simulink model "NMPChighFidelityTiltingQuadrotor"  (R2022b)
settings: Solver=ode4  StartTime=0.0  StopTime=15  FixedStep=Ts  RelTol=1e-3
InitFcn:
  | run initNMPChighFidelityTiltingQuadrotor.m
values from neighbouring files (symbols this model uses):
  lb = 0    [initNMPChighFidelityTiltingQuadrotor.m]
  lbu = repmat(lbu,1,N)    [initNMPChighFidelityTiltingQuadrotor.m]
  lbx = 0    [initNMPChighFidelityTiltingQuadrotor.m]
  N = 30    [initNMPChighFidelityTiltingQuadrotor.m]
  para = repmat(para0,1,N+1)    [initNMPChighFidelityTiltingQuadrotor.m]
  Ts_st = settings.Ts_st    [initNMPChighFidelityTiltingQuadrotor.m]
  ub = 0    [initNMPChighFidelityTiltingQuadrotor.m]
  ubu = repmat(ubu,1,N)    [initNMPChighFidelityTiltingQuadrotor.m]
  ubx = 0    [initNMPChighFidelityTiltingQuadrotor.m]
  W = repmat([Qp Qeq Qv Qomega Qalpha Qw_bar2 Qup Qdotalpha]',1, N)    [initNMPChighFidelityTiltingQuadrotor.m]
  WN = [Qp Qeq Qv Qomega Qalpha Qw_bar2]'    [initNMPChighFidelityTiltingQuadrotor.m]
  z0 = 0    [initNMPChighFidelityTiltingQuadrotor.m]
undefined symbols (not defined in the file or in its folder): DiscIntNeverNeededParam, opt, prop, rad, s, settings, tiltq
libraries: simulink_extras x3, slpidlib x2, aerolibconvert2 x1, robotcorelib x1, uavutilslib x1
settings Model: PauseTimes=2  Creator=chen  LastModifiedBy=beniamino
settings SolverCC: AlgebraicLoopSolver=TrustRegion
settings DataIOCC: ReturnWorkspaceOutputs=off
settings DebuggingCC: UnconnectedInputMsg=warning  UnconnectedOutputMsg=warning  UnconnectedLineMsg=warning  SFMachineParentedDataDiag=warning  ArithmeticOperatorsInVariantConditions=warning
settings ModelReferenceCC: EnableRefExpFcnMdlSchedulingChecks=on
settings SFSimCC: SimUseLocalCustomCode=off  CustomCodeUndefinedFunction=UseInterfaceOnly
settings RTWCC: RTWUseLocalCustomCode=off  CheckMdlBeforeBuild=Error

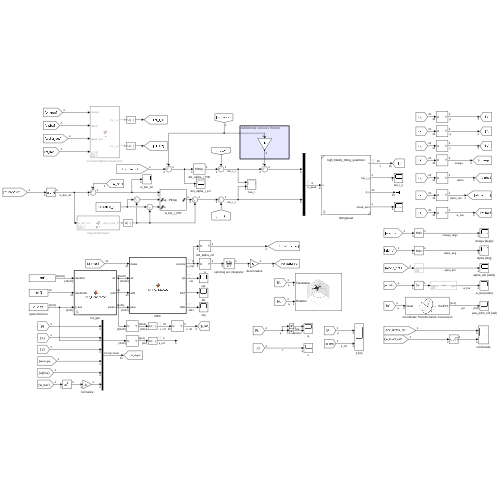
[thumbnail: Simulink's stored preview of the top-level diagram]
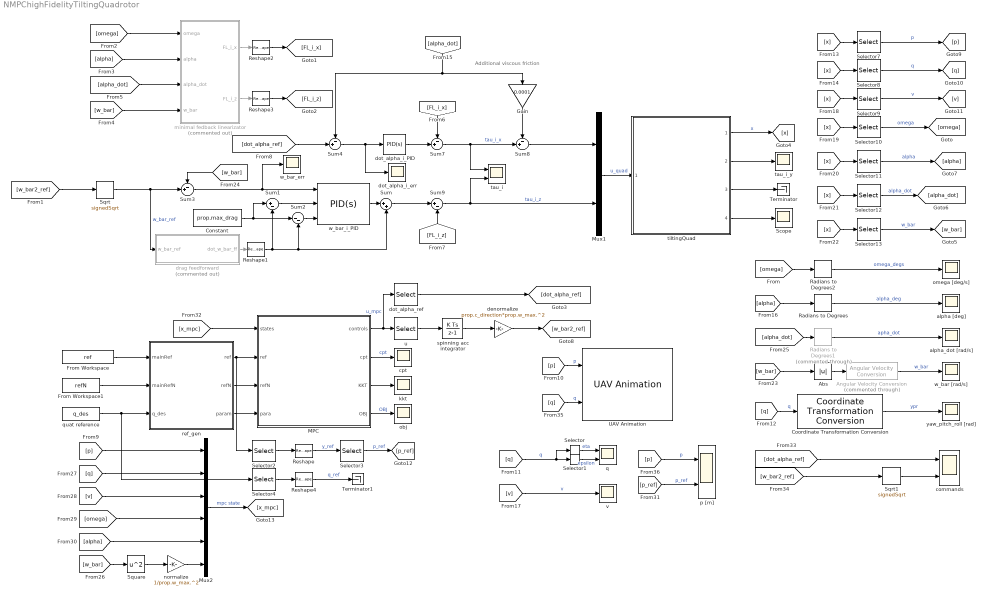
== system NMPChighFidelityTiltingQuadrotor ==
  note: Additional viscous friction
  Abs : Abs  SaturateOnIntegerOverflow=off
  Angular Velocity Conversion : aerolibconvert2/Angular Velocity Conversion  Commented=through  IU=rad/s  OU=rpm
  Constant : Constant  Value=prop.max_drag
  Coordinate Transformation Conversion : robotcorelib/Coordinate Transformation Conversion  InputRepresentation=Quaternion  InputEulerSequence=ZYX  ShowTrVecInputPort=on  OutputRepresentation=Euler Angles  OutputEulerSequence=ZYX  ShowTrVecOutputPort=on  SimulateUsing=Code generation
  From Workspace : FromWorkspace  VariableName=ref  SampleTime=Ts_st  Interpolate=off  OutputAfterFinalValue=Holding final value
  From Workspace1 : FromWorkspace  VariableName=refN  SampleTime=Ts_st  Interpolate=off  OutputAfterFinalValue=Holding final value
  Gain : Gain  Gain=0.0001
  MPC : MATLAB Function  TreatAsAtomicUnit=on
  Mux1 : Mux  Inputs=2
  Mux2 : Mux  Inputs=6
  Radians to Degrees : simulink_extras/Transformations/Radians to Degrees
  Radians to Degrees1 : simulink_extras/Transformations/Radians to Degrees  Commented=through
  Radians to Degrees2 : simulink_extras/Transformations/Radians to Degrees
  Reshape{,1..4} (5 alike) : Reshape
  Scope : Scope
  Selector : Selector  InputPortWidth=4  IndexOptions=Index vector (dialog)  Indices=1  OutputSizes=1
  Selector1 : Selector  InputPortWidth=4  IndexOptions=Index vector (dialog)  Indices=2:4  OutputSizes=1
  Selector10 : Selector  InputPortWidth=25  IndexOptions=Index vector (dialog)  Indices=11:13  OutputSizes=1
  Selector11 : Selector  InputPortWidth=25  IndexOptions=Index vector (dialog)  Indices=14:17  OutputSizes=1
  Selector12 : Selector  InputPortWidth=25  IndexOptions=Index vector (dialog)  Indices=18:21  OutputSizes=1
  Selector13 : Selector  InputPortWidth=25  IndexOptions=Index vector (dialog)  Indices=22:25  OutputSizes=1
  Selector2 : Selector  NumberOfDimensions=2  InputPortWidth=[27 N]  IndexOptions=Select all,Index vector (dialog)  Indices=1:3,1  OutputSizes=1,1
  Selector3 : Selector  InputPortWidth=28  IndexOptions=Index vector (dialog)  Indices=1:3  OutputSizes=1
  Selector4 : Selector  NumberOfDimensions=2  InputPortWidth=[27 N]  IndexOptions=Select all,Index vector (dialog)  Indices=1:3,1  OutputSizes=1,1
  Selector7 : Selector  InputPortWidth=25  IndexOptions=Index vector (dialog)  Indices=1:3  OutputSizes=1
  Selector8 : Selector  InputPortWidth=25  IndexOptions=Index vector (dialog)  Indices=4:7  OutputSizes=1
  Selector9 : Selector  InputPortWidth=25  IndexOptions=Index vector (dialog)  Indices=8:10  OutputSizes=1
  Sqrt : Sqrt  Operator=signedSqrt
  Sqrt1 : Sqrt  Operator=signedSqrt
  Square : Math  Operator=square
  Sum : Sum  Inputs=|++
  Sum1 : Sum  Inputs=|+-
  Sum2 : Sum  Inputs=|--
  Sum{3..4,7..8} (4 alike) : Sum  Inputs=-+|
  Sum9 : Sum  Inputs=|+-
  Terminator : Terminator
  Terminator1 : Terminator
  UAV Animation : uavutilslib/UAV Animation  UAVType=Multirotor  UAVSize=1  InertialZDirection=Up  SampleTime=0.02
  alpha [deg] : Scope
  alpha_dot [rad/s] : Scope
  commands : Scope  NumInputPorts=2
  cpt : Scope
  denormalize : Gain  Gain=prop.c_direction*prop.w_max.^2
  dot_alpha_i_PID : slpidlib/PID Controller  Controller=PID  Form=Parallel  TimeDomain=Continuous-time  UseExternalTs=off  SampleTime=-1  IntegratorMethod=Forward Euler  FilterMethod=Forward Euler  ControllerParametersSource=internal  P=0.01  I=0.1  UseKiTs=off  D=0.00001  N=100  UseFilter=on  TunerSelectOption=Transfer Function Based (PID Tuner App)  InitialConditionSource=internal  InitialConditionForIntegrator=0  InitialConditionForFilter=0  DifferentiatorICPrevScaledInput=0  ExternalReset=none  TrackingMode=off  Kt=1  LimitOutput=off  SatLimitsSource=internal  UpperSaturationLimit=inf  LowerSaturationLimit=-inf  LinearizeAsGain=on  AntiWindupMode=none  Kb=1  LimitIntegrator=off  UpperIntegratorSaturationLimit=inf  LowerIntegratorSaturationLimit=-inf  POutMin=[]  POutMax=[]  IOutMin=[]  IOutMax=[]  DOutMin=[]  DOutMax=[]  NOutMin=[]  NOutMax=[]  SumOutMin=[]  SumOutMax=[]  SaturationOutMin=[]  SaturationOutMax=[]  PParamMin=[]  PParamMax=[]  IParamMin=[]  IParamMax=[]  DParamMin=[]  DParamMax=[]  NParamMin=[]  NParamMax=[]  KbParamMin=[]  KbParamMax=[]  KtParamMin=[]  KtParamMax=[]  KbOutMin=[]  KbOutMax=[]  KtOutMin=[]  KtOutMax=[]  IntegratorOutMin=[]  IntegratorOutMax=[]  FilterOutMin=[]  FilterOutMax=[]  SumI1OutMin=[]  SumI1OutMax=[]  SumI2OutMin=[]  SumI2OutMax=[]  SumI3OutMin=[]  SumI3OutMax=[]  SumI4OutMin=[]  SumI4OutMax=[]  SumDOutMin=[]  SumDOutMax=[]  DifferentiatorOutMin=[]  DifferentiatorOutMax=[]  FilterDiffOutCoefMin=[]  FilterDiffOutCoefMax=[]  ReciprocalOutMin=[]  ReciprocalOutMax=[]  SumDenOutMin=[]  SumDenOutMax=[]  SumNumOutMin=[]  SumNumOutMax=[]  DivideOutMin=[]  DivideOutMax=[]  UdiffTsProdOutMin=[]  UdiffTsProdOutMax=[]  NTsProdOutMin=[]  NTsProdOutMax=[]  UintegralTsProdOutMin=[]  UintegralTsProdOutMax=[]  UngainTsProdOutMin=[]  UngainTsProdOutMax=[]  ClampingZeroOutDataTypeStr=Inherit: Inherit via back propagation  ClampingZeroOutMin=[]  ClampingZeroOutMax=[]  FilterDenConstantOutDataTypeStr=Inherit: Inherit via back propagation  FilterDenConstantOutMin=[]  FilterDenConstantOutMax=[]  PCopyOutDataTypeStr=Inherit: Inherit via back propagation  PCopyOutMin=[]  PCopyOutMax=[]  NCopyOutDataTypeStr=Inherit: Inherit via back propagation  NCopyOutMin=[]  NCopyOutMax=[]  IntegratorContinuousStateAttributes=''  IntegratorStateMustResolveToSignalObject=off  IntegratorRTWStateStorageClass=Auto  FilterContinuousStateAttributes=''  FilterStateMustResolveToSignalObject=off  FilterRTWStateStorageClass=Auto  ParallelPVariant=InternalParameters  IdealPVariant=Disabled  IVariant=InternalParameters  DVariant=InternalParameters  IntegratorVariant=Continuous  SatVariant=Disabled  AWVariant=Passthrough  PCopyVariant=Disabled  TRVariant=Disabled  FdbkBlocksVariant=Forward  IdealPFdbkVariant=Disabled  SatFdbkVariant=Disabled  DerivativeFilterVariant=ContFilter  NVariant=InternalParameters  NCopyVariant=Disabled  FilterICVariant=InternalICsFilter  IntegratorICVariant=InternalICs  ExternalResetVariant=Disabled  TRSumVariant=Passthrough  SumFdbkVariant=Disabled  SumVariant=Sum_PID  TsampFilterVariant=InternalTs  TsampNgainVariant=Passthrough  TsampIntegralVariant=Passthrough  ExternalSaturationOutDataTypeStr=Inherit: Same as second input
  dot_alpha_i_err : Scope
  dot_alpha_ref : Selector  InputPortWidth=8  IndexOptions=Index vector (dialog)  Indices=5:8  OutputSizes=1
  drag feedforward : MATLAB Function  Commented=on  TreatAsAtomicUnit=on  mask{k_m=prop.k_m}
      mask prompts: k_m "motor drag constant"
  kkt : Scope
  minimal fedback linearizator : MATLAB Function  Commented=on  TreatAsAtomicUnit=on  mask{N=tiltq.N, I_i=tiltq.I_i, beta=tiltq.beta}
      mask prompts: N "number of propellers"; I_i "propeller + rotor inertia matrix"; beta "propeller tilting planes angles"
  normalize : Gain  Gain=1/prop.w_max.^2
  obj : Scope
  omega [deg/s] : Scope
  p [m] : Scope  NumInputPorts=2
  q : Scope  NumInputPorts=2
  quat reference : FromWorkspace  VariableName=q_des  SampleTime=Ts_st  Interpolate=off  OutputAfterFinalValue=Holding final value
  ref_gen : MATLAB Function  TreatAsAtomicUnit=on  mask{opt=opt}
      mask prompts: opt "Simulations options structure"
  spinning acc integrator : DiscreteIntegrator  InitialCondition=0.33*ones(4,1)  SampleTime=-1  ICPrevOutput=DiscIntNeverNeededParam  ICPrevScaledInput=DiscIntNeverNeededParam
  tau_i : Scope  NumInputPorts=2
  tau_i_y : Scope
  tiltingQuad : Subsystem  ReferencedSubsystem=high_fidelity_tilting_quadrotor  p0=p_0  q0=q_0  v0=v_0  omega0=omega_0  alpha0=alpha_0  d_alpha_0=alpha_dot_0  bar_w0=w_bar_0  m_b=tiltq.m_b  beta=tiltq.beta  I_b=body.I  I_i=tiltq.I_i  c_direction=prop.c_direction  k_m=prop.k_m  k_t=prop.k_t  p_mot=tiltq.p_mot  min_alpha=tiltq.min_alpha  max_alpha=tiltq.max_alpha  min_d_alpha=tiltq.min_alpha_dot  max_d_alpha=tiltq.max_alpha_dot  min_bar_w=[prop.w_min prop.w_min -prop.w_max -prop.w_max]  max_bar_w=[prop.w_max prop.w_max -prop.w_min -prop.w_min]
  u : Selector  InputPortWidth=8  IndexOptions=Index vector (dialog)  Indices=1:4  OutputSizes=1
  v : Scope
  w_bar [rad/s] : Scope
  w_bar_err : Scope
  w_bar_i_PID : slpidlib/PID Controller  Controller=PID  Form=Parallel  TimeDomain=Continuous-time  UseExternalTs=off  SampleTime=-1  IntegratorMethod=Forward Euler  FilterMethod=Forward Euler  ControllerParametersSource=internal  P=0.01  I=0.1  UseKiTs=on  D=0.00001  N=100  UseFilter=on  TunerSelectOption=Transfer Function Based (PID Tuner App)  InitialConditionSource=internal  InitialConditionForIntegrator=0  InitialConditionForFilter=0  DifferentiatorICPrevScaledInput=0  ExternalReset=none  TrackingMode=off  Kt=1  LimitOutput=on  SatLimitsSource=external  UpperSaturationLimit=inf  LowerSaturationLimit=-inf  LinearizeAsGain=on  AntiWindupMode=back-calculation  Kb=10  LimitIntegrator=off  UpperIntegratorSaturationLimit=inf  LowerIntegratorSaturationLimit=-inf  POutMin=[]  POutMax=[]  IOutMin=[]  IOutMax=[]  DOutMin=[]  DOutMax=[]  NOutMin=[]  NOutMax=[]  SumOutMin=[]  SumOutMax=[]  SaturationOutMin=[]  SaturationOutMax=[]  PParamMin=[]  PParamMax=[]  IParamMin=[]  IParamMax=[]  DParamMin=[]  DParamMax=[]  NParamMin=[]  NParamMax=[]  KbParamMin=[]  KbParamMax=[]  KtParamMin=[]  KtParamMax=[]  KbOutMin=[]  KbOutMax=[]  KtOutMin=[]  KtOutMax=[]  IntegratorOutMin=[]  IntegratorOutMax=[]  FilterOutMin=[]  FilterOutMax=[]  SumI1OutMin=[]  SumI1OutMax=[]  SumI2OutMin=[]  SumI2OutMax=[]  SumI3OutMin=[]  SumI3OutMax=[]  SumI4OutMin=[]  SumI4OutMax=[]  SumDOutMin=[]  SumDOutMax=[]  DifferentiatorOutMin=[]  DifferentiatorOutMax=[]  FilterDiffOutCoefMin=[]  FilterDiffOutCoefMax=[]  ReciprocalOutMin=[]  ReciprocalOutMax=[]  SumDenOutMin=[]  SumDenOutMax=[]  SumNumOutMin=[]  SumNumOutMax=[]  DivideOutMin=[]  DivideOutMax=[]  UdiffTsProdOutMin=[]  UdiffTsProdOutMax=[]  NTsProdOutMin=[]  NTsProdOutMax=[]  UintegralTsProdOutMin=[]  UintegralTsProdOutMax=[]  UngainTsProdOutMin=[]  UngainTsProdOutMax=[]  ClampingZeroOutDataTypeStr=Inherit: Inherit via back propagation  ClampingZeroOutMin=[]  ClampingZeroOutMax=[]  FilterDenConstantOutDataTypeStr=Inherit: Inherit via back propagation  FilterDenConstantOutMin=[]  FilterDenConstantOutMax=[]  PCopyOutDataTypeStr=Inherit: Inherit via back propagation  PCopyOutMin=[]  PCopyOutMax=[]  NCopyOutDataTypeStr=Inherit: Inherit via back propagation  NCopyOutMin=[]  NCopyOutMax=[]  IntegratorContinuousStateAttributes=''  IntegratorStateMustResolveToSignalObject=off  IntegratorRTWStateStorageClass=Auto  FilterContinuousStateAttributes=''  FilterStateMustResolveToSignalObject=off  FilterRTWStateStorageClass=Auto  ParallelPVariant=InternalParameters  IdealPVariant=Disabled  IVariant=InternalParameters  DVariant=InternalParameters  IntegratorVariant=Continuous  SatVariant=External  AWVariant=BackCalculation  PCopyVariant=Disabled  TRVariant=Disabled  FdbkBlocksVariant=Forward  IdealPFdbkVariant=Disabled  SatFdbkVariant=Disabled  DerivativeFilterVariant=ContFilter  NVariant=InternalParameters  NCopyVariant=Disabled  FilterICVariant=InternalICsFilter  IntegratorICVariant=InternalICs  ExternalResetVariant=Disabled  TRSumVariant=Passthrough  SumFdbkVariant=Disabled  SumVariant=Sum_PID  TsampFilterVariant=InternalTs  TsampNgainVariant=Passthrough  TsampIntegralVariant=Passthrough  ExternalSaturationOutDataTypeStr=Inherit: Same as second input
  yaw_pitch_roll [rad] : Scope
  wires:
  MPC/1(controls) -> u/1, dot_alpha_ref/1  "u_mpc"
  MPC/2(cpt) -> cpt/1  "cpt"
  MPC/4(OBJ) -> obj/1  "OBJ"
  MPC/3(KKT) -> kkt/1
  ref_gen/1(ref) -> Selector2/1, MPC/2(ref)
  ref_gen/2(refN) -> MPC/3(refN)
  [alpha_dot] -> Sum4/1, Gain/1
  Mux1/1 -> tiltingQuad/1  "u_quad"
  Sum2/1 -> w_bar_i_PID/3
  [w_bar] -> minimal fedback linearizator/4(w_bar)
  Reshape1/1 -> Sum/2, Sum2/2, Sum1/2
  Gain/1 -> Sum8/1
  tiltingQuad/3 -> Terminator/1
  [w_bar] -> Sum3/1
  minimal fedback linearizator/1(FL_i_x) -> Reshape2/1
  tiltingQuad/1 -> [x]  "x"
  tiltingQuad/2 -> tau_i_y/1
  Sum7/1 -> tau_i/1, Sum8/2  "tau_i_x"
  Sum1/1 -> w_bar_i_PID/2
  [omega] -> minimal fedback linearizator/1(omega)
  Sum9/1 -> Mux1/2, tau_i/2  "tau_i_z"
  [w_bar2_ref] -> Sqrt/1
  [FL_i_x] -> Sum7/1
  [FL_i_z] -> Sum9/2
  w_bar_i_PID/1 -> Sum/1
  Constant/1 -> Sum2/1, Sum1/1
  [alpha_dot] -> minimal fedback linearizator/3(alpha_dot)
  tiltingQuad/4 -> Scope/1
  Sum4/1 -> dot_alpha_i_err/1, dot_alpha_i_PID/1
  [alpha] -> minimal fedback linearizator/2(alpha)
  minimal fedback linearizator/2(FL_i_z) -> Reshape3/1
  Sum8/1 -> Mux1/1
  Sum/1 -> Sum9/1
  Sqrt/1 -> Sum3/2, drag feedforward/1(w_bar_ref)  "w_bar_ref"
  dot_alpha_i_PID/1 -> Sum7/2
  [x] -> Selector10/1
  Selector11/1 -> [alpha]  "alpha"
  Selector12/1 -> [alpha_dot]  "alpha_dot"
  Selector10/1 -> [omega]  "omega"
  [x] -> Selector13/1
  Selector13/1 -> [w_bar]  "w_bar"
  [x] -> Selector12/1
  [x] -> Selector11/1
  [alpha] -> Radians to Degrees/1
  Selector1/1 -> q/2  "epsilon"
  Radians to Degrees/1 -> alpha [deg]/1  "alpha_deg"
  [q] -> Selector1/1, Selector/1  "q"
  Radians to Degrees2/1 -> omega [deg/s]/1  "omega_degs"
  Radians to Degrees1/1 -> alpha_dot [rad/s]/1  "apha_dot"
  [w_bar] -> Abs/1
  Angular Velocity Conversion/1 -> w_bar [rad/s]/1  "w_bar"
  [x] -> Selector9/1
  Abs/1 -> Angular Velocity Conversion/1
  [x] -> Selector8/1
  [alpha_dot] -> Radians to Degrees1/1
  [p] -> UAV Animation/1  "p"
  Selector/1 -> q/1  "eta"
  [omega] -> Radians to Degrees2/1
  [v] -> v/1  "v"
  [x] -> Selector7/1
  dot_alpha_ref/1 -> [dot_alpha_ref]
  u/1 -> spinning acc integrator/1
  denormalize/1 -> [w_bar2_ref]
  [dot_alpha_ref] -> Sum4/2
  Sqrt1/1 -> commands/2
  Coordinate Transformation Conversion/1 -> yaw_pitch_roll [rad]/1  "ypr"
  Mux2/1 -> [x_mpc]  "mpc state"
  [w_bar] -> Square/1
  Square/1 -> normalize/1
  normalize/1 -> Mux2/6
  Sum3/1 -> w_bar_err/1, w_bar_i_PID/1
  spinning acc integrator/1 -> denormalize/1
  Selector7/1 -> [p]  "p"
  Selector8/1 -> [q]  "q"
  [q] -> Coordinate Transformation Conversion/1  "q"
  Selector9/1 -> [v]  "v"
  [alpha] -> Mux2/5
  [omega] -> Mux2/4
  [v] -> Mux2/3
  [q] -> Mux2/2
  [p] -> Mux2/1
  From Workspace/1 -> ref_gen/1(mainRef)
  From Workspace1/1 -> ref_gen/2(mainRefN)
  quat reference/1 -> Selector4/1, ref_gen/3(q_des)
  ref_gen/3(param) -> MPC/4(para)
  Selector2/1 -> Reshape/1
  [p_ref] -> p [m]/2  "p_ref"
  Reshape/1 -> Selector3/1  "y_ref"
  drag feedforward/1(dot_w_bar_ff) -> Reshape1/1
  Reshape2/1 -> [FL_i_x]
  Reshape3/1 -> [FL_i_z]
  [x_mpc] -> MPC/1(states)
  [w_bar2_ref] -> Sqrt1/1
  [dot_alpha_ref] -> commands/1
  [q] -> UAV Animation/2  "q"
  [p] -> p [m]/1  "p"
  Selector3/1 -> [p_ref]  "p_ref"
  Selector4/1 -> Reshape4/1
  Reshape4/1 -> Terminator1/1  "q_ref"

== matlab function NMPChighFidelityTiltingQuadrotor/ref_gen ==
  data: ref output; settings parameter; refN output; mainRef input; opt parameter; mainRefN input; q_des input; param output; para parameter
function [ref,refN, param] = Ref_Generator(settings, mainRef, opt, mainRefN, q_des, para)

switch opt.ref_type
    case 0
        p_ref = [1 1 1];
        qe_ref = [0 0 0];
        v_ref = [0 0 0];
        omega_ref = [0 0 0];
        alpha_ref = [0 0 0 0];
        w_bar_ref = 0.33*ones(1,4);
        u_ref = [0 0 0 0];
        dot_alpha_ref = [0 0 0 0];
        REF=[p_ref qe_ref v_ref omega_ref alpha_ref w_bar_ref u_ref dot_alpha_ref];
        ref = repmat(REF',1,settings.N);
        refN = REF(1:settings.nyN)';
        param = para;
    case 2
        ref = mainRef;
        refN = mainRefN;
        param =  q_des;
    otherwise
        p_ref = [0 0 0];
        qe_ref = [0 0 0];
        v_ref = [0 0 0];
        omega_ref = [0 0 0];
        alpha_ref = [0 0 0 0];
        w_bar_ref = 0.33*ones(1,4);
        u_ref = [0 0 0 0];
        dot_alpha_ref = [0 0 0 0];
        REF=[p_ref qe_ref v_ref omega_ref alpha_ref w_bar_ref u_ref dot_alpha_ref];
        ref = repmat(REF',1,settings.N);
        refN = REF(1:settings.nyN)';
        param = para;
end


%     ref = repmat([1.4, 0, 0]',1,settings.N);
%     refN = 1.4;

== matlab function NMPChighFidelityTiltingQuadrotor/minimal fedback linearizator ==
  data: omega input; alpha input; FL_i_x output; beta parameter; N parameter; alpha_dot input; w_bar input; FL_i_z output; I_i parameter
function [FL_i_x, FL_i_z]= fcn(omega, alpha, beta, N, alpha_dot, w_bar, I_i)

FL_i_x = zeros(4,1);
FL_i_z = zeros(4,1);

for i=1:N
    B_R_i = axang2rotm([0 0 1 beta(i)])*axang2rotm([1 0 0 alpha(i)]);
    omega_i = B_R_i.' * omega + [alpha_dot(i); 0; w_bar(i)];
    coriol_i = cross(omega_i, I_i*omega_i);
    FF_i = coriol_i;
    FL_i_x(i) = -FF_i(1);
    FL_i_z(i) = -FF_i(3);
end

== matlab function NMPChighFidelityTiltingQuadrotor/drag feedforward ==
  data: w_bar_ref input; dot_w_bar_ff output; k_m parameter
function dot_w_bar_ff = fcn(w_bar_ref, k_m)

dot_w_bar_ff = k_m .* w_bar_ref .* abs(w_bar_ref);

== matlab function NMPChighFidelityTiltingQuadrotor/MPC ==
  settings: updateMethod=DISCRETE  sampleTime=Ts_st
  data: states input size=nx; settings parameter; opt parameter; lb parameter; ub parameter; lbx parameter; ubx parameter; lbu parameter; ubu parameter; W parameter; WN parameter; ref input size=[ny N]; refN input size=nyN; z0 parameter; controls output size=nu; cpt output size=1; KKT output; OBJ output; para input
function [controls, cpt, KKT, OBJ] = NMPC_BLOCK(states, settings, opt, lb, ub, lbx, ubx, lbu, ubu, W, WN, ref, refN, z0, para)

%% everything should has a fixed size
coder.extrinsic('mpc_nmpcsolver_simulink');  
coder.extrinsic('InitData');  
coder.extrinsic('InitMemory');  
coder.extrinsic('evalin');
coder.extrinsic('assignin');

%%

persistent x u z lambda mu mu_x mu_u;
persistent input mem;

if isempty(input)  
    
    nx = settings.nx;        % No. of differential states
    nu = settings.nu;        % No. of controls
    nz = settings.nz;        % No. of algebraic states
    ny = settings.ny;        % No. of outputs (references)    
    nyN= settings.nyN;       % No. of outputs at terminal stage 
    np = settings.np;        % No. of parameters (on-line data)
    nc = settings.nc;        % No. of constraints
    ncN = settings.ncN;      % No. of constraints at terminal stage
    nbu = settings.nbu;      % No. of control bounds
    nbx = settings.nbx;      % No. of state bounds
    nbu_idx = settings.nbu_idx; % Index of control bounds
    nbx_idx = settings.nbx_idx; % Index of state bounds
    N = settings.N;
    N2 = settings.N2;
    r = settings.r;
        
    input.x0=states;
    
    x=repmat(states,1,N+1);
    input.x=x;
    
    u=zeros(nu,N);
    input.u=u;
    
    z=repmat(z0,1,N);
    input.z=z;
    
    lambda = zeros(nx,N+1);
    input.lambda= lambda;
    
    if N*nc+ncN > 0
        mu = zeros(N*nc+ncN,1);
    else
        mu = 0;
    end
    input.mu= mu;
    
    mu_u = zeros(N*nu,1);
    input.mu_u= mu_u;
    
    if N*nbx > 0
        mu_x = zeros(N*nbx,1);
    else
        mu_x = 0;
    end
    input.mu_x = mu_x;
    
    input.W=W;
    input.WN=WN;
    input.od = para;
    
    input.lb = lb;
    input.ub = ub;
    input.lbx = lbx;
    input.ubx = ubx;
    input.lbu = lbu;
    input.ubu = ubu;
      
    input.y = ref;
    input.yN = refN;
    
    mem = InitMemory(settings, opt, input);
        
else

    input.x=x; 
    input.u=u;
    input.z=z;
    input.lambda=lambda;   
    input.mu=mu;
    input.mu_x=mu_x;
    input.mu_u=mu_u;

    input.y = ref;
    input.yN = refN;
    
end

%%
cpt = 0;
KKT = 0;
OBJ = 0;
input.x0 = states;
[input,mem,cpt,KKT,OBJ] = mpc_nmpcsolver_simulink(input, settings, mem, opt);
controls = input.u(:,1);

%% shifting
switch opt.shifting
    case 'yes'
        x=[input.x(:,2:end),input.x(:,end)];  
        u=[input.u(:,2:end),input.u(:,end)]; 
        z=[input.z(:,2:end),input.z(:,end)]; 
        lambda=[input.lambda(:,2:end),input.lambda(:,end)];
        if (settings.N*settings.nc+settings.ncN) >0
            mu(1:end-settings.ncN+1)=input.mu(settings.nc+1:settings.N*settings.nc+settings.ncN,1);
            mu(settings.N*settings.nc+1:end)=input.mu(settings.N*settings.nc+settings.ncN-settings.nc+1:settings.N*settings.nc+settings.ncN,1);
        else
            mu=0;
        end
        mu_x=[input.mu_x(2:end,1);input.mu_x(end,1)];
        mu_u=[input.mu_u(2:end,1);input.mu_u(end,1)];
   case 'no'
        x=input.x;
        u=input.u;
        z=input.z;
        lambda=input.lambda;
        mu=input.mu;
        mu_x=input.mu_x;
        mu_u=input.mu_u;
end

return
